simulink model "FPGA_SMC"  (R2019b)
settings: Solver=FixedStepAuto  StartTime=0.0  StopTime=10.0  RelTol=1e-3
undefined symbols (not defined in the file): DiscIntNeverNeededParam
settings Model: SILPILModeSetting=veronly  ExtModeTrigDuration=2  Creator=Anas  LastModifiedBy=Anas
settings OptimizationCC: BlockReduction=off  ConditionallyExecuteInputs=off  DefaultParameterBehavior=Inlined  UseFloatMulNetSlope=on  DefaultUnderspecifiedDataType=single  EnhancedBackFolding=on  PassReuseOutputArgsAs=Individual arguments  ZeroExternalMemoryAtStartup=off  ZeroInternalMemoryAtStartup=off  MaxStackSize=64  OptimizeBlockOrder=speed  DifferentSizesBufferReuse=on  OptimizationCustomize=off  EfficientTunableParamExpr=on
settings DebuggingCC: AlgebraicLoopMsg=error  ParameterTunabilityLossMsg=error
settings HardwareCC: ProdBitPerPointer=32  ProdBitPerSizeT=32  ProdBitPerPtrDiffT=32  ProdLargestAtomicFloat=None  ProdIntDivRoundTo=Undefined  ProdEndianess=Unspecified  ProdWordSize=32  ProdHWDeviceType=ASIC/FPGA->ASIC/FPGA  TargetBitPerPointer=64  TargetBitPerSizeT=64  TargetBitPerPtrDiffT=64  TargetLongLongMode=on  TargetIntDivRoundTo=Zero  TargetEndianess=LittleEndian  TargetWordSize=64  TargetHWDeviceType=Custom Processor->MATLAB Host Computer  ProdEqTarget=off  HardwareBoardFeatureSet=SoCBlockset
settings SFSimCC: MATLABDynamicMemAlloc=off
settings RTWCC: SystemTargetFile=ert.tlc  HardwareBoard=Custom Hardware Board  TLCOptions="-aInlineSetEventsForThisBaseRateFcn=TLC_FALSE -aSuppressMultiTaskScheduler=TLC_FALSE  -aRateBasedStepFcn=0"  TemplateMakefile=ert_default_tmf  GenerateReport=on  BuildConfiguration=Faster Runs  IncludeHyperlinkInReport=on  LaunchReport=on  GenerateTraceInfo=on  GenerateTraceReport=on  GenerateTraceReportSl=on  GenerateTraceReportSf=on  GenerateTraceReportEml=on
settings CodeAppCC: ForceParamTrailComments=on  IgnoreCustomStorageClasses=off  OperatorAnnotations=on  SimulinkDataObjDesc=on  SFDataObjDesc=on  InsertBlockDesc=on
settings ERTTargetCC: InlinedParameterPlacement=NonHierarchical

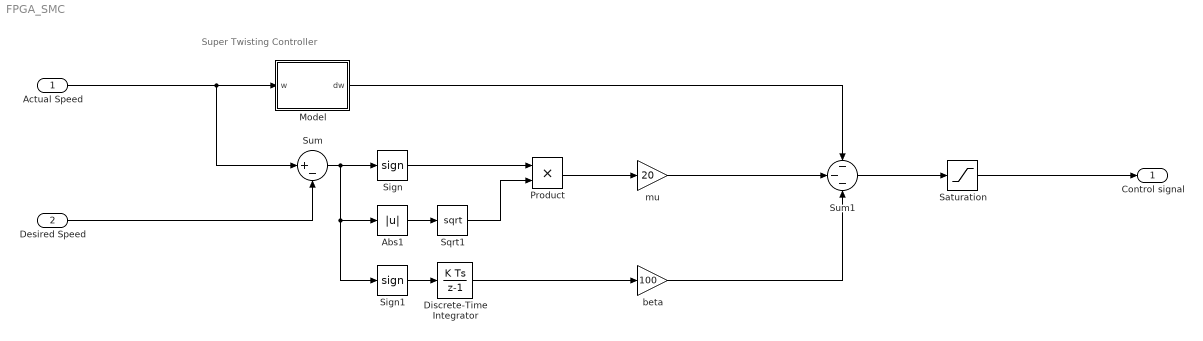
== system FPGA_SMC ==
  note: Super Twisting Controller
  Actual Speed : Inport
  Desired Speed : Inport  Port=2
  Abs1 : Abs
  Discrete-Time Integrator : DiscreteIntegrator  SampleTime=-1  OutDataTypeStr=single  ICPrevOutput=DiscIntNeverNeededParam  ICPrevScaledInput=DiscIntNeverNeededParam
  Model : MATLAB Function  TreatAsAtomicUnit=on
  Product : Product
  Saturation : Saturate  UpperLimit=5  LowerLimit=-5
  Sign : Signum
  Sign1 : Signum
  Sqrt1 : Sqrt  IntermediateResultsDataTypeStr=double  SaturateOnIntegerOverflow=on
  Sum : Sum  Inputs=|+-
  Sum1 : Sum  Inputs=---
  beta : Gain  Gain=100
  mu : Gain  Gain=20
  "Control signal " : Outport  VectorParamsAs1DForOutWhenUnconnected=off
  wires:
  Saturation/1 -> "Control signal "/1
  Sqrt1/1 -> Product/2
  Abs1/1 -> Sqrt1/1
  Desired Speed/1 -> Sum/2
  Sign/1 -> Product/1
  Sum/1 -> Abs1/1, Sign1/1, Sign/1
  Model/1(dw) -> Sum1/1
  Sign1/1 -> Discrete-Time Integrator/1
  beta/1 -> Sum1/3
  Discrete-Time Integrator/1 -> beta/1
  Actual Speed/1 -> Sum/1, Model/1(w)
  mu/1 -> Sum1/2
  Product/1 -> mu/1
  Sum1/1 -> Saturation/1

== matlab function FPGA_SMC/Model ==
  data: w input; dw output
function dw = Model(w)
%System Model
dw=-0.08653*w^2-39.902*w;
end
